simulink model "AC_Voltage_Controller_eight"  (R2020a)
settings: Solver=ode23tb  StartTime=0.0  StopTime=0.1  MinStep=1e-6  RelTol=1e-6
libraries: powerlib x13, powerlib_meascontrol x2
settings Model: Creator=Siddharthan A  LastModifiedBy=ASUS
settings SolverCC: ZeroCrossControl=DisableAll

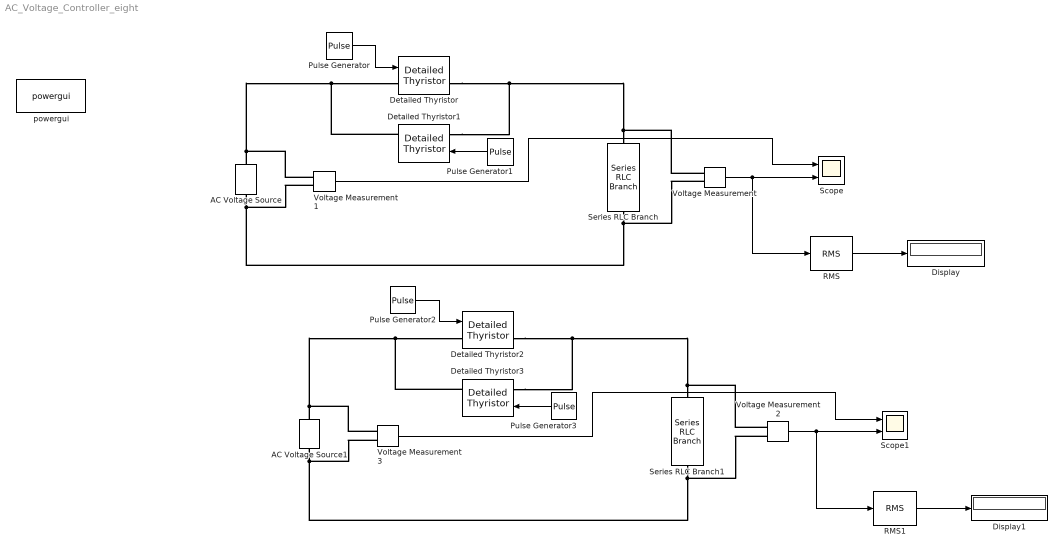
== system AC_Voltage_Controller_eight ==
  AC Voltage Source : powerlib/Electrical Sources/AC Voltage Source  Amplitude=24*sqrt(2)  Phase=0  Frequency=50  SampleTime=0  Measurements=None  BusType=swing  Pref=10e3  Qref=0  Qmin=-inf  Qmax=+inf
  AC Voltage Source1 : powerlib/Electrical Sources/AC Voltage Source  Amplitude=24*sqrt(2)  Phase=0  Frequency=50  SampleTime=0  Measurements=None  BusType=swing  Pref=10e3  Qref=0  Qmin=-inf  Qmax=+inf
  Detailed Thyristor{,1..3} (4 alike) : powerlib/Power Electronics/Detailed Thyristor  Ron=0.001  Lon=1e-3  Vf=0.8  IL=0.1  Tq=100e-6  IC=0  Rs=500  Cs=250e-9  Measurements=on
      settings: SourceProductBaseCode=PS
  Display : Display
  Display1 : Display
  Pulse Generator : DiscretePulseGenerator  PulseType=Time based  Period=0.02  PulseWidth=50  PhaseDelay=(0.01/180)*90
  Pulse Generator1 : DiscretePulseGenerator  PulseType=Time based  Period=0.02  PulseWidth=50  PhaseDelay=0.01+(0.01/180)*(90)
  Pulse Generator2 : DiscretePulseGenerator  PulseType=Time based  Period=0.02  PulseWidth=50  PhaseDelay=(0.01/180)*45
  Pulse Generator3 : DiscretePulseGenerator  PulseType=Time based  Period=0.02  PulseWidth=50  PhaseDelay=0.01+(0.01/180)*(45)
  RMS : powerlib_meascontrol/Measurements/RMS  TrueRMS=on  Freq=60  RMSInit=120  Ts=0
  RMS1 : powerlib_meascontrol/Measurements/RMS  TrueRMS=on  Freq=60  RMSInit=120  Ts=0
  Scope : Scope  NumInputPorts=2
  Scope1 : Scope  NumInputPorts=2
  Series RLC Branch : powerlib/Elements/Series RLC Branch  LConnTagsString=__new0  RConnTagsString=__new0  BranchType=R  Resistance=10  Inductance=1e-3  SetiL0=off  InitialCurrent=0  Capacitance=1e-6  Setx0=off  InitialVoltage=0  Measurements=None
  Series RLC Branch1 : powerlib/Elements/Series RLC Branch  LConnTagsString=__new0  RConnTagsString=__new0  BranchType=RL  Resistance=10  Inductance=6600e-6  SetiL0=off  InitialCurrent=0  Capacitance=1e-6  Setx0=off  InitialVoltage=0  Measurements=None
  Voltage Measurement{,1..3} (4 alike) : powerlib/Measurements/Voltage Measurement  PhasorSimulation=off  OutputType=Complex  PSBequivalent=0
  powergui : powerlib/powergui  Priority=1  SimulationMode=Continuous  SampleTime=50e-6  frequency=60  Iterations=50  frequencyindice=0  Pbase=100e6  ErrMax=1e-4  UnitsV=kV  UnitsW=MW  buscounter=0  FunctionMessages=off  echomessages=off  EnableUseOfTLC=off  CurrentSourceSwitches=off  DisableSnubberDevices=off  DisableRonSwitches=off  DisableVfSwitches=off  DisplayEquations=off  AutomaticDiscreteSolvers=off  SolverType=Tustin/Backward Euler (TBE)  Interpol=off  ExternalGateDelay=off  methode=off  Ts=100  x0status=blocks  SPID=on  SwTol=0  HookPort=off  NonlinearTolerance=1e-4  nMaxIteration=100  ContinueOnMaxIteration=off  RestoreLinks=warning  ResistiveCurrentMeasurement=off  Frange=[0:2:500]  Ylog=off  Xlog=on  ShowGrid=off  save=off  variable=ZData  structure=0  ZoomFFT=off  StartTime=0.0  cycles=1  DisplayStyle=1  fundamental=60  FreqAxis=off  MaxFrequency=1000  frequencyindicesteady=1  RmsSteady=1  display=off
  wires:
  Voltage Measurement/1 -> RMS/1, Scope/2
  Voltage Measurement1/1 -> Scope/1
  Pulse Generator1/1 -> Detailed Thyristor1/1
  Pulse Generator/1 -> Detailed Thyristor/1
  RMS/1 -> Display/1
  RMS1/1 -> Display1/1
  Pulse Generator2/1 -> Detailed Thyristor2/1
  Pulse Generator3/1 -> Detailed Thyristor3/1
  Voltage Measurement3/1 -> Scope1/1
  Voltage Measurement2/1 -> Scope1/2, RMS1/1
  connections:
  AC Voltage Source/RConn1 -- Voltage Measurement1/LConn1 -- Detailed Thyristor1/RConn1 -- Detailed Thyristor/LConn1
  Detailed Thyristor/RConn1 -- Detailed Thyristor1/LConn1 -- Voltage Measurement/LConn1 -- Series RLC Branch/LConn1
  Series RLC Branch/RConn1 -- Voltage Measurement/LConn2 -- Voltage Measurement1/LConn2 -- AC Voltage Source/LConn1
  AC Voltage Source1/RConn1 -- Detailed Thyristor2/LConn1 -- Detailed Thyristor3/RConn1 -- Voltage Measurement3/LConn1
  Detailed Thyristor2/RConn1 -- Series RLC Branch1/LConn1 -- Voltage Measurement2/LConn1 -- Detailed Thyristor3/LConn1
  Series RLC Branch1/RConn1 -- AC Voltage Source1/LConn1 -- Voltage Measurement3/LConn2 -- Voltage Measurement2/LConn2
